simulink model "PTODi"  (R2018a)
settings: configuration reference "cs_ert" (kept outside this file)
settings Model: DataDictionary=PTODi.sldd  Creator=zhoutinglin  LastModifiedBy=zhoutinglin

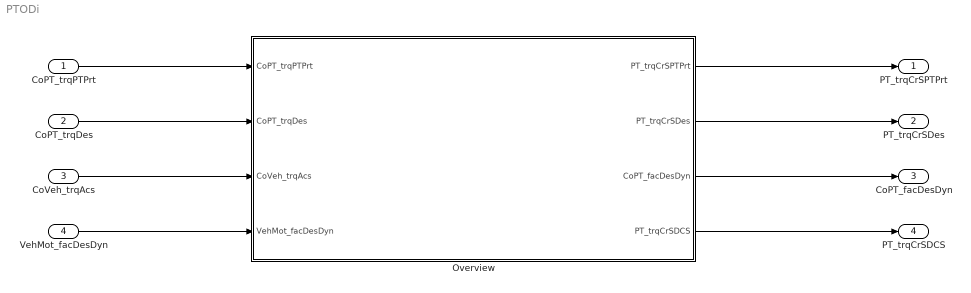
== system PTODi ==
  CoPT_trqPTPrt : Inport
  CoPT_trqDes : Inport  Port=2
  CoVeh_trqAcs : Inport  Port=3
  VehMot_facDesDyn : Inport  Port=4
  Overview : Subsystem
  PT_trqCrSPTPrt : Outport
  PT_trqCrSDes : Outport  Port=2
  CoPT_facDesDyn : Outport  Port=3
  PT_trqCrSDCS : Outport  Port=4
  wires:
  CoPT_trqPTPrt/1 -> Overview/1(CoPT_trqPTPrt)
  CoPT_trqDes/1 -> Overview/2(CoPT_trqDes)
  CoVeh_trqAcs/1 -> Overview/3(CoVeh_trqAcs)
  VehMot_facDesDyn/1 -> Overview/4(VehMot_facDesDyn)
  Overview/1(PT_trqCrSPTPrt) -> PT_trqCrSPTPrt/1
  Overview/2(PT_trqCrSDes) -> PT_trqCrSDes/1
  Overview/3(CoPT_facDesDyn) -> CoPT_facDesDyn/1
  Overview/4(PT_trqCrSDCS) -> PT_trqCrSDCS/1

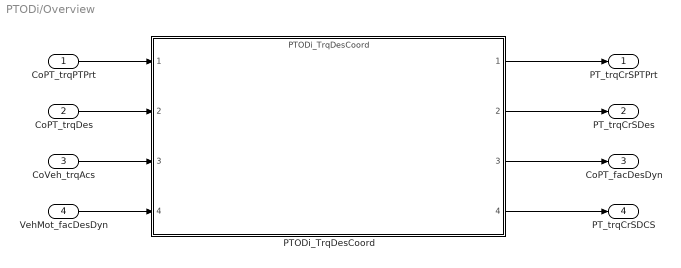
== system PTODi/Overview ==
  CoPT_trqPTPrt : Inport
  CoPT_trqDes : Inport  Port=2
  CoVeh_trqAcs : Inport  Port=3
  VehMot_facDesDyn : Inport  Port=4
  PTODi_TrqDesCoord : ModelReference  ModelNameDialog=PTODi_TrqDesCoord  SimulationMode=Normal  ModelReferenceVersion=1.49
  PT_trqCrSPTPrt : Outport
  PT_trqCrSDes : Outport  Port=2
  CoPT_facDesDyn : Outport  Port=3
  PT_trqCrSDCS : Outport  Port=4
  wires:
  CoPT_trqPTPrt/1 -> PTODi_TrqDesCoord/1
  CoPT_trqDes/1 -> PTODi_TrqDesCoord/2
  CoVeh_trqAcs/1 -> PTODi_TrqDesCoord/3
  VehMot_facDesDyn/1 -> PTODi_TrqDesCoord/4
  PTODi_TrqDesCoord/1 -> PT_trqCrSPTPrt/1
  PTODi_TrqDesCoord/2 -> PT_trqCrSDes/1
  PTODi_TrqDesCoord/3 -> CoPT_facDesDyn/1
  PTODi_TrqDesCoord/4 -> PT_trqCrSDCS/1
